simulink library "GFL_Lib"  (R2017a)
settings: Solver=VariableStepAuto  StartTime=0.0  StopTime=10.0  RelTol=1e-3
values from neighbouring files (symbols this model uses):
  Va0 = Vm0*sqrt(2)*Vb1*sin(Theta_Vm0*pi/180)    [Init_LF_L.m]
  Vb0 = Vm0*sqrt(2)*Vb1*sin(Theta_Vm0*pi/180-2*pi/3)    [Init_LF_L.m]
  Vc0 = Vm0*sqrt(2)*Vb1*sin(Theta_Vm0*pi/180+2*pi/3)    [Init_LF_L.m]
  Vm0 = abs(V1)    [Init_LF_L.m]
  Vm0_d = Vvsc0*cos(angle(Vvirt))    [Init_LF_L.m]
  Vm0_q = Vvsc0*sin(angle(Vvirt))    [Init_LF_L.m]
  Vvsc0 = abs(Vvirt)    [Init_LF_L.m]
undefined symbols (not defined in the file or in its folder): Diff_CC_ki, Diff_CC_kp, fb, Ib2, Idcb, Ki_i, Ki_Wdiff_pu, Ki_Wtot_pu, Kp_i, Kp_Rvi_pu, Kp_Wdiff_pu, Kp_Wtot_pu, Lb, Lc_eq, Lc_pu, Lf_pu, Sb, Solver_Time_Step, Vb1, Vb2, Vdcb, VSC01_id0, wb, Zb
undefined symbols (not defined in the file): Carm, Time_Step
libraries: powerlib x90, Control_Lib x57, spsCurrentMeasurementLib x7, simulink x7, spsControlledCurrentSourceLib x6, GFL_Lib x5, Source_Lib x2, eeGeneralControl x2, powerlib_meascontrol x2, GFo_Lib x1
(part 1 of 5)
settings Model: Creator=Frederic_Colas  LastModifiedBy=Frederic_Colas

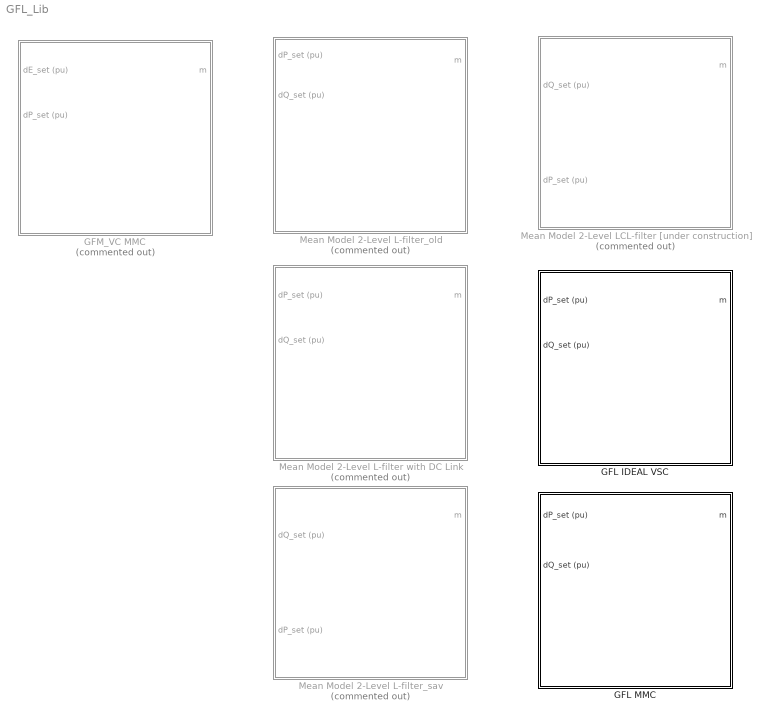
== system GFL_Lib ==
  GFL IDEAL VSC : Subsystem  mask(VSC){fn=50, Sn=1000e6, Pn=1000e6, Udcn=640e3, Output_Delay=100e-6, Un1=320e3, Un2=400e3, m=1, Rt_pu=0.005, Lt_pu=0.15+0.18/2, Lm_pu=500, Rm_pu=500, DC_Link=Perfect DC Source, H_DC=inf, H_DC_sav=inf, wn_PLL=50, zeta_PLL=1, QV=Voltage Control, w_P=5, w_V=10, w_LPF=30, wn_i=4000, zeta_i=1, Kffi=on, Filtre_FF=off, w_ff=4000, Imax=5, Iqmax=5, K_FRT=0, Advanced=on, LFpopup=PQ, P0=0, Q0=0, V0=1, Theta0=0}
      mask prompts: fn "Nominal Frequency (Hz)"; Sn "Nominal Apparent Power (VA)"; Pn "Nominal Power (W)"; Udcn "Nominal DC Voltage (V)"; Output_Delay "Equivalent Ouput Delay (s)"; Un1 "VSC side Nominal Ph-Ph Voltage (V)"; Un2 "Grid side Nominal Ph-Ph Voltage (V)"; m "Transformer's ratio (p.u)"; Rt_pu "R (pu)"; Lt_pu "L (pu)"; Lm_pu "Rm (pu)"; Rm_pu "Lm (pu)"; H_DC "DC Inertia (ms)"; wn_PLL "Bandwidth (rad/s)"; zeta_PLL "Damping Ratio"; QV "Mode"; w_P "Power control bandwidth (rad/s)"; w_V "Voltage control bandwidth (rad/s)"; w_LPF "Low-pass filters bandwidth (rad/s)"; wn_i "Bandwidth (rad/s)"; zeta_i "Damping factor"; Kffi "Feedfoward Enable"; Filtre_FF "Filter of ff enable"; w_ff "Cutoff pulsation (rad/s)"; Imax "Maximum current"; Iqmax "Maximum quadrature current"; K_FRT "LVRT block enabled (1) or disabled (0)"; P0 "Initial Active Power (pu)"; Q0 "Initial Reactive Power (pu)"; V0 "Initial Voltage (pu)"; Theta0 "Initial Angle (°)"
      mask init:
      | Init_Base;
      | dLc_pu = 0;
      | Init_VI;
      | Init_LF_L;
      | Init_GFL;
      settings: OpenFcn=|
      | NameStr = get_param(gcb,'Name');
      | open_system(gcbh, 'Mask');
      | 
      | h2AllOpenDlgs = DAStudio.ToolRoot.getOpenDialogs;
      | 
      | for i=1:length(h2AllOpenDlgs)
      |     try
      |          %disp(h2AllOpenDlgs(i).getSource.getBlock.Name);
      |         Dialog_block_name = h2AllOpenDlgs(i).getSource.getBlock.Name;
      |          %strcmp(Dialog_block_name, NameStr),
      |         if (strcmp(h2AllOpenDlgs(i).getSource.getBlock.Name, NameStr))
      |             iPos = h2AllOpenDlgs(i).position;
      |             h2AllOpenDlgs(i).position = [iPos(1)   iPos(2)   iPos(3)*1.4   iPos(4)];
      |         end
      |     end
      | end
      mask TypeOptions DC_Link: Perfect DC Source | No DC link capacitor | DC link capacitor
      mask Callback DC_Link:
      | % Get the mask parameter values. This is a cell
      | %   array of character vectors.
      | maskStr = get_param(gcb,'DC_Link');
      | p=Simulink.Mask.get(gcb);
      | 
      | % The pop-up menu is the first mask parameter.
      | %   Check the value selected in the pop-up
      | if strcmp(maskStr,'Perfect DC Source'),
      |     % Set the visibility of both parameters on when
      |     %   User-defined is selected in the pop-up.
      |     if strcmp(p.getParameter('H_DC').Visible,'on')
      |         p.getParameter('H_DC_sav').Value=p.getParameter('H_DC').Value;
      |     end
      |     p.getParameter('H_DC').Visible='off';
      |     p.getParameter('H_DC').Value='inf';
      | elseif strcmp(maskStr,'No DC link capacitor'),
      |     if strcmp(p.getParameter('H_DC').Visible,'on')
      |         p.getParameter('H_DC_sav').Value=p.getParameter('H_DC').Value;
      |     end
      |     p.getParameter('H_DC').Visible='off';
      |     p.getParameter('H_DC').Value='0';
      | else
      |     % Set the visibility of both parameters on when
      |     %   User-defined is selected in the pop-up.
      |     p.getParameter('H_DC').Visible='on';
      |     p.getParameter('H_DC').Value=p.getParameter('H_DC_sav').Value;
      | end
      mask TypeOptions QV: Voltage Control | Reactive Power Control
      mask Callback Advanced:
      | % Get the mask parameter values. This is a cell
      | %   array of character vectors.
      | maskStr = get_param(gcb,'Advanced');
      | p=Simulink.Mask.get(gcb);
      | 
      | % The pop-up menu is the first mask parameter.
      | %   Check the value selected in the pop-up
      | if strcmp(maskStr,'on'),
      | 
      |     % Set the visibility of both parameters on when
      |     %   User-defined is selected in the pop-up.
      |     p.getDialogControl('Current_Loop').Visible='on';
      |     %p.getDialogControl('TVI').Visible='on';
      |     %p.getDialogControl('LC_Filter').Visible='on';
      |     p.getDialogControl('Current_Sat').Visible='on';
      |     p.getDialogControl('LVRT').Visible='on';
      | 
      | 
      | else
      | 
      |     % Set the visibility of both parameters on when
      |     %   User-defined is selected in the pop-up.
      |     p.getDialogControl('Current_Loop').Visible='off';
      |     %p.getDialogControl('TVI').Visible='on';
      |     %p.getDialogControl('LC_Filter').Visible='on';
      |     p.getDialogControl('Current_Sat').Visible='off';
      |     p.getDialogControl('LVRT').Visible='off';
      | 
      | end
      mask TypeOptions LFpopup: Swing | PQ | PV
      mask Callback LFpopup:
      | % Get the mask parameter values. This is a cell
      | %   array of character vectors.
      | maskStr = get_param(gcb,'LFpopup');
      | p=Simulink.Mask.get(gcb);
      | 
      | % The pop-up menu is the first mask parameter.
      | %   Check the value selected in the pop-up
      | if strcmp(maskStr,'Swing'),
      | 
      |     % Set the visibility of both parameters on when
      |     %   User-defined is selected in the pop-up.
      |     p.getParameter('P0').Visible='off';
      |     p.getParameter('Q0').Visible='off';
      |     p.getParameter('V0').Visible='on';
      |     p.getParameter('Theta0').Visible='on';
      |     set_param([gcb '/Source_For_LF'],'BusType','swing');
      | 
      | elseif strcmp(maskStr,'PQ'),
      | 
      |     % Set the visibility of both parameters on when
      |     %   User-defined is selected in the pop-up.
      |     p.getParameter('P0').Visible='on';
      |     p.getParameter('Q0').Visible='on';
      |     p.getParameter('V0').Visible='off';
      |     p.getParameter('Theta0').Visible='off';
      |     set_param([gcb '/Source_For_LF'],'BusType','PQ');
      | 
      |     % Turn off the visibility of the Value field
      |     %   when User-defined is not selected.
      | else
      | 
      |     % Set the visibility of both parameters on when
      |     %   User-defined is selected in the pop-up.
      |     p.getParameter('P0').Visible='on';
      |     p.getParameter('Q0').Visible='off';
      |     p.getParameter('V0').Visible='on';
      |     p.getParameter('Theta0').Visible='off';
      |     set_param([gcb '/Source_For_LF'],'BusType','PV');
      | 
      | end
      mask DialogControl Container13 Prompt: PLL
      mask DialogControl Container11 Prompt: Outer loop
      mask DialogControl Current_Loop Prompt: Current Loop
      mask DialogControl Current_Sat Prompt: Current saturations
      mask DialogControl LVRT Prompt: LVRT
      mask DialogControl Control4 Prompt: Initial Operating Point
      mask DialogControl Container24 Prompt: VSC side
      mask DialogControl LF_vsc_str Prompt: V0 = 1.0002 pu, Angle = 0.013461°
      mask DialogControl Container25 Prompt: PCC
      mask DialogControl UpdateLoadflow Prompt: Update Loadflow
      mask DialogControl UpdateLoadflow Callback: LoadFlow_VSC
      mask Display:
      | x1=0.05;
      | y1=0.2;
      | %
      | plot([0.5 0.5]+x1,[0.97,0.8]-y1)
      | plot([0.5 0.32]+x1,[0.80 0.71]-y1)
      | plot([0.32 0.32]+x1,[0.80 0.52]-y1)
      | plot([0.32 0.5]+x1,[0.62 0.52]-y1)
      | plot([0.5 0.5]+x1,[0.52 0.35]-y1)
      | plot([0.45 0.5 0.43]+x1,[0.59 0.52 0.51]-y1)
      | %
      | plot([0.28 0.28]+x1,[0.74 0.58]-y1)
      | plot([0.28 0.20]+x1,[0.66 0.66]-y1)
      | %
      | plot([0.5 0.63]+x1,[0.84 0.84]-y1)
      | plot([0.63 0.63]+x1,[0.84 0.72]-y1)
      | plot([0.63 0.59]+x1,[0.72 0.65]-y1)
      | plot([0.63 0.67]+x1,[0.72 0.65]-y1)
      | plot([0.59 0.67]+x1,[0.65 0.65]-y1)
      | plot([0.63 0.63]+x1,[0.65 0.47]-y1)
      | plot([0.5 0.63]+x1,[0.47 0.47]-y1)
      | plot([0.58 0.67]+x1,[0.72 0.72]-y1)
      | %
      | color('blue')
      | text(0.3,0.10,'L-Filter GFL')
      | 
      | port_label('input',1,'\DeltaP (pu)','texmode','on');
      | port_label('input',2,'\DeltaQ (pu)','texmode','on');
      | port_label('output',1,'m');
      | port_label('rconn',1,'A');
      | port_label('rconn',2,'B');
      | port_label('rconn',3,'C');
      | port_label('lconn',1,'+');
      | port_label('lconn',2,'-');
  GFL MMC : Subsystem  mask(VSC){fn=50, Sn=1e9, Pn=1e9, Udcn=640e3, Output_Delay=100e-6, Un1=320e3, Un2=400e3, m=1, Rt_pu=0.005, Lt_pu=0.15, Lm_pu=500, Rm_pu=500, Larm_pu=0.18, Rarm_pu=0.005, nSM=0, Hc=40, wn_PLL=50, zeta_PLL=1, QV=Voltage Control, w_P=5, w_V=50, w_LPF=1000, wn_i=300, zeta_i=1, Kffi=on, Filtre_FF=on, w_ff=4000, Imax=5, Iqmax=5, K_FRT=0, MMC_Control_Type=CCSC, Diff_CC_fn=0, Diff_CC_zeta=0, fn_Wtot=0, zeta_Wtot=0, fn_Wdiff=0, zeta_Wdiff=0, Advanced=off, LFpopup=PQ, P0=0, Q0=0, V0=1, Theta0=0}
      mask prompts: fn "Nominal Frequency (Hz)"; Sn "Nominal Apparent Power (VA)"; Pn "Nominal Power (W)"; Udcn "Nominal DC Voltage (V)"; Output_Delay "Equivalent Ouput Delay (s)"; Un1 "VSC side Nominal Ph-Ph Voltage (V)"; Un2 "Grid side Nominal Ph-Ph Voltage (V)"; m "Transformer's ratio (p.u)"; Rt_pu "R (pu)"; Lt_pu "L (pu)"; Lm_pu "Rm (pu)"; Rm_pu "Lm (pu)"; Larm_pu "Arm Inductance (pu)"; Rarm_pu "Arm Resistance (pu)"; nSM "Sub-Modules number"; Hc "Hc (ms)"; wn_PLL "Bandwidth (rad/s)"; zeta_PLL "Damping Ratio"; QV "Mode"; w_P "Power control bandwidth (rad/s)"; w_V "Voltage control bandwidth (rad/s)"; w_LPF "Low-pass filters bandwidth (rad/s)"; wn_i "Bandwidth (rad/s)"; zeta_i "Damping factor"; Kffi "Feedfoward Enable"; Filtre_FF "Filter of ff enable"; w_ff "Cutoff frequency (rad/s)"; Imax "Maximum current"; Iqmax "Maximum quadrature current"; K_FRT "LVRT block enabled (1) or disabled (0)"; MMC_Control_Type "Controller Type"; Diff_CC_fn "Bandwidth (Hz)"; Diff_CC_zeta "Damping"; fn_Wtot "Bandwidth (Hz)"; zeta_Wtot "Damping"; fn_Wdiff "Bandwidth (Hz)"; zeta_Wdiff "Damping"; P0 "Initial Active Power (pu)"; Q0 "Initial Reactive Power (pu)"; V0 "Initial Voltage (pu)"; Theta0 "Initial Angle (°)"
      mask init:
      | Init_Base;
      | dLc_pu = 0;
      | Init_VI_mmc;
      | Init_MMC;
      | Init_LF_MMC;
      | Init_GFL;
      settings: OpenFcn=|
      | NameStr = get_param(gcb,'Name');
      | open_system(gcbh, 'Mask');
      | 
      | h2AllOpenDlgs = DAStudio.ToolRoot.getOpenDialogs;
      | 
      | for i=1:length(h2AllOpenDlgs)
      |     try
      |          %disp(h2AllOpenDlgs(i).getSource.getBlock.Name);
      |         Dialog_block_name = h2AllOpenDlgs(i).getSource.getBlock.Name;
      |          %strcmp(Dialog_block_name, NameStr),
      |         if (strcmp(h2AllOpenDlgs(i).getSource.getBlock.Name, NameStr))
      |             iPos = h2AllOpenDlgs(i).position;
      |             h2AllOpenDlgs(i).position = [iPos(1)   iPos(2)   iPos(3)*1.4   iPos(4)];
      |         end
      |     end
      | end
      mask TypeOptions QV: Voltage Control | Reactive Power Control
      mask TypeOptions MMC_Control_Type: CCSC | Energy Based
      mask Callback MMC_Control_Type:
      | % Get the mask parameter values. This is a cell
      | %   array of character vectors.
      | maskStr = get_param(gcb,'MMC_Control_Type');
      | p=Simulink.Mask.get(gcb);
      | 
      | % The pop-up menu is the first mask parameter.
      | %   Check the value selected in the pop-up
      | if strcmp(maskStr,'CCSC'),
      | 
      |     % Set the visibility of both parameters on when
      |     %   User-defined is selected in the pop-up.
      |     p.getDialogControl('Diff_CC').Visible='on';
      |     %p.getDialogControl('TVI').Visible='on';
      |     %p.getDialogControl('LC_Filter').Visible='on';
      |     p.getDialogControl('Wtot_C').Visible='off';
      |     p.getDialogControl('Wdiff_C').Visible='off';
      |     %p.getDialogControl('Param_Strat_3').Visible='off';
      | 
      | 
      | else
      | 
      |     % Set the visibility of both parameters on when
      |     %   User-defined is selected in the pop-up.
      |     p.getDialogControl('Diff_CC').Visible='on';
      |     %p.getDialogControl('TVI').Visible='on';
      |     %p.getDialogControl('LC_Filter').Visible='on';
      |     p.getDialogControl('Wtot_C').Visible='on';
      |     p.getDialogControl('Wdiff_C').Visible='on';
      |     %p.getDialogControl('Param_Strat_3').Visible='off';
      | 
      | end
      mask Callback Advanced:
      | % Get the mask parameter values. This is a cell
      | %   array of character vectors.
      | maskStr = get_param(gcb,'Advanced');
      | p=Simulink.Mask.get(gcb);
      | 
      | % The pop-up menu is the first mask parameter.
      | %   Check the value selected in the pop-up
      | if strcmp(maskStr,'on'),
      | 
      |     % Set the visibility of both parameters on when
      |     %   User-defined is selected in the pop-up.
      |     p.getDialogControl('Current_Loop').Visible='on';
      |     %p.getDialogControl('TVI').Visible='on';
      |     %p.getDialogControl('LC_Filter').Visible='on';
      |     p.getDialogControl('Current_Sat').Visible='on';
      |     p.getDialogControl('LVRT').Visible='on';
      |     p.getDialogControl('MMC_Control').Visible='on';
      | 
      | 
      | else
      | 
      |     % Set the visibility of both parameters on when
      |     %   User-defined is selected in the pop-up.
      |     p.getDialogControl('Current_Loop').Visible='off';
      |     %p.getDialogControl('TVI').Visible='on';
      |     %p.getDialogControl('LC_Filter').Visible='on';
      |     p.getDialogControl('Current_Sat').Visible='off';
      |     p.getDialogControl('LVRT').Visible='off';
      |     p.getDialogControl('MMC_Control').Visible='off';
      | 
      | end
      mask TypeOptions LFpopup: Swing | PQ | PV
      mask Callback LFpopup:
      | % Get the mask parameter values. This is a cell
      | %   array of character vectors.
      | maskStr = get_param(gcb,'LFpopup');
      | p=Simulink.Mask.get(gcb);
      | 
      | % The pop-up menu is the first mask parameter.
      | %   Check the value selected in the pop-up
      | if strcmp(maskStr,'Swing'),
      | 
      |     % Set the visibility of both parameters on when
      |     %   User-defined is selected in the pop-up.
      |     p.getParameter('P0').Visible='off';
      |     p.getParameter('Q0').Visible='off';
      |     p.getParameter('V0').Visible='on';
      |     p.getParameter('Theta0').Visible='on';
      |     set_param([gcb '/Source_For_LF'],'BusType','swing');
      | 
      | elseif strcmp(maskStr,'PQ'),
      | 
      |     % Set the visibility of both parameters on when
      |     %   User-defined is selected in the pop-up.
      |     p.getParameter('P0').Visible='on';
      |     p.getParameter('Q0').Visible='on';
      |     p.getParameter('V0').Visible='off';
      |     p.getParameter('Theta0').Visible='off';
      |     set_param([gcb '/Source_For_LF'],'BusType','PQ');
      | 
      |     % Turn off the visibility of the Value field
      |     %   when User-defined is not selected.
      | else
      | 
      |     % Set the visibility of both parameters on when
      |     %   User-defined is selected in the pop-up.
      |     p.getParameter('P0').Visible='on';
      |     p.getParameter('Q0').Visible='off';
      |     p.getParameter('V0').Visible='on';
      |     p.getParameter('Theta0').Visible='off';
      |     set_param([gcb '/Source_For_LF'],'BusType','PV');
      | 
      | end
      mask DialogControl Container13 Prompt: PLL
      mask DialogControl Container11 Prompt: Outer loop
      mask DialogControl Current_Loop Prompt: Current Loop
      mask DialogControl Current_Sat Prompt: Current saturations
      mask DialogControl LVRT Prompt: LVRT
      mask DialogControl MMC_Control Prompt: MMC Controller
      mask DialogControl Diff_CC Prompt: Differential Current Controller
      mask DialogControl Wtot_C Prompt: Wtot Controller
      mask DialogControl Wdiff_C Prompt: Wdiff Controller
      mask DialogControl Control4 Prompt: Initial Operating Point
      mask DialogControl Container24 Prompt: VSC side
      mask DialogControl LF_vsc_str Prompt: V0 = 1.0003 pu, Angle = 0.018328°
      mask DialogControl Container25 Prompt: PCC
      mask DialogControl UpdateLoadflow Prompt: Update Loadflow
      mask DialogControl UpdateLoadflow Callback: LoadFlow_VSC
      mask Display:
      | % Q1
      | x1=-0.07;
      | y1=+0.03;
      | plot([0.4 0.4]+x1,[0.90,0.80]+y1)
      | plot([0.4 0.33]+x1,[0.80 0.74]+y1)
      | plot([0.33 0.33]+x1,[0.78 0.66]+y1)
      | plot([0.33 0.4]+x1,[0.70 0.64]+y1)
      | plot([0.4 0.4]+x1,[0.64 0.55]+y1)
      | plot([0.38 0.40 0.35]+x1,[0.68 0.64 0.64]+y1)
      | plot([0.30 0.30]+x1,[0.74 0.7]+y1)
      | plot([0.29 0.27]+x1,[0.72 0.72]+y1)
      | % Q2
      | y1=y1-0.51;
      | plot([0.4 0.4]+x1,[0.90,0.80]+y1)
      | plot([0.4 0.33]+x1,[0.80 0.74]+y1)
      | plot([0.33 0.33]+x1,[0.78 0.66]+y1)
      | plot([0.33 0.4]+x1,[0.70 0.64]+y1)
      | plot([0.4 0.4]+x1,[0.64 0.55]+y1)
      | plot([0.39 0.40 0.35]+x1,[0.68 0.64 0.64]+y1)
      | plot([0.30 0.30]+x1,[0.75 0.7]+y1)
      | plot([0.29 0.27]+x1,[0.72 0.72]+y1)
      | % Q3
      | y1=y1+0.51;
      | x1=x1+0.22+0.1;
      | plot([0.4 0.4]+x1,[0.90,0.80]+y1)
      | plot([0.4 0.33]+x1,[0.80 0.74]+y1)
      | plot([0.33 0.33]+x1,[0.78 0.66]+y1)
      | plot([0.33 0.4]+x1,[0.70 0.64]+y1)
      | plot([0.4 0.4]+x1,[0.64 0.55]+y1)
      | plot([0.39 0.41 0.34]+x1,[0.68 0.64 0.64]+y1)
      | plot([0.30 0.30]+x1,[0.75 0.7]+y1)
      | plot([0.29 0.27]+x1,[0.72 0.72]+y1)
      | % Q4
      | y1=y1-0.51;
      | x1=x1;
      | plot([0.4 0.4]+x1,[0.90,0.80]+y1)
      | plot([0.4 0.33]+x1,[0.80 0.74]+y1)
      | plot([0.33 0.33]+x1,[0.78 0.66]+y1)
      | plot([0.33 0.4]+x1,[0.70 0.64]+y1)
      | plot([0.4 0.4]+x1,[0.64 0.55]+y1)
      | plot([0.39 0.41 0.34]+x1,[0.68 0.64 0.64]+y1)
      | plot([0.30 0.30]+x1,[0.75 0.7]+y1)
      | plot([0.29 0.26]+x1,[0.72 0.72]+y1)
      | %
      | x1=-0.05;
      | y1=+0.03;
      | plot([0.90 0.40]+x1,[0.9 0.9]+y1)
      | plot([0.90 0.40]+x1,[0.04 0.04]+y1)
      | %
      | 
      | plot([0.69 0.42]+x1,[0.4 0.4]+y1)
      | plot([0.38 0.22]+x1,[0.52 0.52]+y1)
      | plot([0.22 0.22]+x1,[0.52 0.54]+y1)
      | plot([0.22 0.22]+x1,[0.56 0.58]+y1)
      | plot([0.22 0.22]+x1,[0.60 0.63]+y1)
      | %
      | plot([0.35 0.22]+x1,[0.4 0.4]+y1)
      | plot([0.22 0.22]+x1,[0.4 0.37]+y1)
      | plot([0.22 0.22]+x1,[0.4 0.37]+y1)
      | plot([0.22 0.22]+x1,[0.35 0.32]+y1)
      | plot([0.22 0.22]+x1,[0.30 0.27]+y1)
      | %
      | plot([0.38 0.38]+x1,[ 0.55 0.38]+y1)
      | plot([0.7 0.7]+x1,[0.55 0.3]+y1)
      | %
      | % D1
      | x1=-0.07;
      | y1=+0.03;
      | plot([0.4 0.45]+x1,[0.84,0.84]+y1)
      | plot([0.45 0.45]+x1,[0.84,0.75]+y1)
      | plot([0.45 0.41]+x1,[0.75,0.72]+y1)
      | plot([0.45 0.48]+x1,[0.75,0.72]+y1)
      | plot([0.41 0.48]+x1,[0.72,0.72]+y1)
      | plot([0.45 0.45]+x1,[0.72,0.6]+y1)
      | plot([0.4 0.45]+x1,[0.6,0.6]+y1)
      | % D2
      | x1=x1+0.22+0.1;
      | plot([0.4 0.45]+x1,[0.84,0.84]+y1)
      | plot([0.45 0.45]+x1,[0.84,0.75]+y1)
      | plot([0.45 0.43]+x1,[0.75,0.72]+y1)
      | plot([0.45 0.48]+x1,[0.75,0.72]+y1)
      | %
      | plot([0.43 0.48]+x1,[0.72,0.72]+y1)
      | plot([0.45 0.45]+x1,[0.72,0.6]+y1)
      | plot([0.4 0.45]+x1,[0.6,0.6]+y1)
      | % D3
      | x1=x1-0.22-0.1;
      | y1=y1-0.5;
      | plot([0.4 0.45]+x1,[0.84,0.84]+y1)
      | plot([0.45 0.45]+x1,[0.84,0.75]+y1)
      | plot([0.45 0.41]+x1,[0.75,0.72]+y1)
      | plot([0.45 0.48]+x1,[0.75,0.72]+y1)
      | plot([0.41 0.48]+x1,[0.72,0.72]+y1)
      | plot([0.45 0.45]+x1,[0.72,0.6]+y1)
      | plot([0.4 0.45]+x1,[0.6,0.6]+y1)
      | % D4
      | x1=x1+0.22+0.1;
      | plot([0.4 0.45]+x1,[0.84,0.84]+y1)
      | plot([0.45 0.45]+x1,[0.84,0.75]+y1)
      | plot([0.45 0.43]+x1,[0.75,0.72]+y1)
      | plot([0.45 0.48]+x1,[0.75,0.72]+y1)
      | plot([0.43 0.48]+x1,[0.72,0.72]+y1)
      | plot([0.45 0.45]+x1,[0.72,0.6]+y1)
      | plot([0.40 0.45]+x1,[0.6,0.6]+y1)
      | color('blue');
      | disp('MMC GFL');
      | port_label('input',1,'\DeltaE (pu)','texmode','on');
      | port_label('input',2,'\DeltaP (pu)','texmode','on');
      | port_label('output',1,'m');
      | port_label('rconn',1,'A');
      | port_label('rconn',2,'B');
      | port_label('rconn',3,'C');
      | port_label('lconn',1,'+');
      | port_label('lconn',2,'-');
  GFM_VC MMC : Subsystem  Commented=on  mask(VSC){fn=50, Sn=1000e6, Pn=1000e6, Udcn=640e3, Output_Delay=100e-6, Un1=320e3, Un2=400e3, Rt_pu=0.005, Lt_pu=0.15, Lm_pu=500, Rm_pu=500, Larm_pu=0.18, Rarm_pu=0.005, nSM=0, Hc=40, DC_source=on, wn_PLL=50, zeta_PLL=1, Val_Freq_Support=off, R_percent=4, dLc_pu=0, Rv=0.009, W_TVR=60, I_max_pu=2, Tr_I_max=10, I_Max_TVI_pu=2, DX_DR=5, MMC_Control_Type=CCSC, Diff_CC_fn=200, Diff_CC_zeta=1, fn_Wtot=3, zeta_Wtot=1, fn_Wdiff=3, zeta_Wdiff=1, Advanced=on, gainpopup=With Inertia, wn_Inertia_Less=5, Param_Inertia=PI, H_GFo=5, zeta_GFo=1, LFpopup=PQ, P0=0, Q0=0, V0=1, Theta0=9.4519e-16}
      mask prompts: fn "Nominal Frequency (Hz)"; Sn "Nominal Apparent Power (VA)"; Pn "Nominal Power (W)"; Udcn "Nominal DC Voltage (V)"; Output_Delay "Equivalent Output Delay (s)"; Un1 "VSC side Nominal Ph-Ph Voltage (V)"; Un2 "Grid side Nominal Ph-Ph Voltage (V)"; Rt_pu "R (pu)"; Lt_pu "L (pu)"; Lm_pu "Rm (pu)"; Rm_pu "Lm (pu)"; Larm_pu "Arm Inductance (pu)"; Rarm_pu "Arm Resistance (pu)"; nSM "Sub-Modules number"; Hc "Hc (ms)"; DC_source "Perfect DC source"; wn_PLL "Bandwidth (rad/s)"; zeta_PLL "Damping Ratio"; Val_Freq_Support "Frequency Support"; R_percent "Droop Gain (%)"; dLc_pu "Additional Virtual Impedance (pu)"; Rv "Damping Resistance (Rv)"; W_TVR "Dr filter"; I_max_pu "I max (pu)"; Tr_I_max "Current Loop time response (ms)"; I_Max_TVI_pu "Current Threshold (pu)"; MMC_Control_Type "Controller Type"; Diff_CC_fn "Bandwidth (Hz)"; Diff_CC_zeta "Damping"; fn_Wtot "Bandwidth (Hz)"; zeta_Wtot "Damping"; fn_Wdiff "Bandwidth (Hz)"; zeta_Wdiff "Damping"; gainpopup "Strategy"; wn_Inertia_Less "Bandwidth (rad/s)"; H_GFo "Inertia H (s)"; zeta_GFo "Damping Ratio"; P0 "Initial Active Power (pu)"; Q0 "Initial Reactive Power (pu)"; V0 "Initial Voltage (pu)"; Theta0 "Initial Angle (°)"
      mask init:
      | Init_Base;
      | Init_VI;
      | Init_MMC;
      | Init_LF_MMC;
      | Init_GFM;
      settings: OpenFcn=|
      | NameStr = get_param(gcb,'Name');
      | open_system(gcbh, 'Mask');
      | 
      | h2AllOpenDlgs = DAStudio.ToolRoot.getOpenDialogs;
      | 
      | for i=1:length(h2AllOpenDlgs)
      |     try
      |          %disp(h2AllOpenDlgs(i).getSource.getBlock.Name);
      |         Dialog_block_name = h2AllOpenDlgs(i).getSource.getBlock.Name;
      |          %strcmp(Dialog_block_name, NameStr),
      |         if (strcmp(h2AllOpenDlgs(i).getSource.getBlock.Name, NameStr))
      |             iPos = h2AllOpenDlgs(i).position;
      |             h2AllOpenDlgs(i).position = [iPos(1)   iPos(2)   iPos(3)*1.4   iPos(4)];
      |         end
      |     end
      | end
      mask TypeOptions MMC_Control_Type: CCSC | Energy Based
      mask Callback MMC_Control_Type:
      | % Get the mask parameter values. This is a cell
      | %   array of character vectors.
      | maskStr = get_param(gcb,'MMC_Control_Type');
      | p=Simulink.Mask.get(gcb);
      | 
      | % The pop-up menu is the first mask parameter.
      | %   Check the value selected in the pop-up
      | if strcmp(maskStr,'CCSC'),
      | 
      |     % Set the visibility of both parameters on when
      |     %   User-defined is selected in the pop-up.
      |     p.getDialogControl('Diff_CC').Visible='on';
      |     %p.getDialogControl('TVI').Visible='on';
      |     %p.getDialogControl('LC_Filter').Visible='on';
      |     p.getDialogControl('Wtot_C').Visible='off';
      |     p.getDialogControl('Wdiff_C').Visible='off';
      |     %p.getDialogControl('Param_Strat_3').Visible='off';
      | 
      | 
      | else
      | 
      |     % Set the visibility of both parameters on when
      |     %   User-defined is selected in the pop-up.
      |     p.getDialogControl('Diff_CC').Visible='on';
      |     %p.getDialogControl('TVI').Visible='on';
      |     %p.getDialogControl('LC_Filter').Visible='on';
      |     p.getDialogControl('Wtot_C').Visible='on';
      |     p.getDialogControl('Wdiff_C').Visible='on';
      |     %p.getDialogControl('Param_Strat_3').Visible='off';
      | 
      | end
      mask Callback Advanced:
      | % Get the mask parameter values. This is a cell
      | %   array of character vectors.
      | maskStr = get_param(gcb,'Advanced');
      | p=Simulink.Mask.get(gcb);
      | 
      | % The pop-up menu is the first mask parameter.
      | %   Check the value selected in the pop-up
      | if strcmp(maskStr,'on'),
      | 
      |     % Set the visibility of both parameters on when
      |     %   User-defined is selected in the pop-up.
      |     p.getDialogControl('TVR').Visible='on';
      |     %p.getDialogControl('TVI').Visible='on';
      |     %p.getDialogControl('LC_Filter').Visible='on';
      |     p.getDialogControl('Current_Sat').Visible='on';
      |     p.getDialogControl('MMC_Control').Visible='on';
      |     %p.getDialogControl('Param_Strat_3').Visible='off';
      | 
      | 
      | else
      | 
      |     % Set the visibility of both parameters on when
      |     %   User-defined is selected in the pop-up.
      |     p.getDialogControl('TVR').Visible='off';
      |     %p.getDialogControl('TVI').Visible='off';
      |     %p.getDialogControl('LC_Filter').Visible='off';
      |     p.getDialogControl('Current_Sat').Visible='off';
      |     p.getDialogControl('MMC_Control').Visible='off';
      |     %p.getDialogControl('Param_Strat_3').Visible='off';
      | 
      | end
      mask TypeOptions gainpopup: Inertia Less | With Inertia
      mask Callback gainpopup:
      | % Get the mask parameter values. This is a cell
      | %   array of character vectors.
      | maskStr = get_param(gcb,'gainpopup');
      | p=Simulink.Mask.get(gcb);
      | 
      | % The pop-up menu is the first mask parameter.
      | %   Check the value selected in the pop-up
      | if strcmp(maskStr,'Inertia Less'),
      | 
      |     % Set the visibility of both parameters on when
      |     %   User-defined is selected in the pop-up.
      |     p.getDialogControl('No_Inertia').Visible='on';
      |     p.getDialogControl('Inertia').Visible='off';
      |     %p.getDialogControl('Param_Strat_3').Visible='off';
      | 
      | 
      | elseif strcmp(maskStr,'With Inertia'),
      | 
      |     % Set the visibility of both parameters on when
      |     %   User-defined is selected in the pop-up.
      |     p.getDialogControl('No_Inertia').Visible='off';
      |     p.getDialogControl('Inertia').Visible='on';
      |     %p.getDialogControl('Param_Strat_3').Visible='off';
      | 
      | 
      |     % Turn off the visibility of the Value field
      |     %   when User-defined is not selected.
      | 
      | else
      | 
      |     % Set the visibility of both parameters on when
      |     %   User-defined is selected in the pop-up.
      |     p.getDialogControl('No_Inertia').Visible='off';
      |     p.getDialogControl('Inertia').Visible='off';
      |     %p.getDialogControl('Param_Strat_3').Visible='off';
      | 
      | end
      mask TypeOptions Param_Inertia: VSM | PI
      mask TypeOptions LFpopup: Swing | PQ | PV
      mask Callback LFpopup:
      | % Get the mask parameter values. This is a cell
      | %   array of character vectors.
      | maskStr = get_param(gcb,'LFpopup');
      | p=Simulink.Mask.get(gcb);
      | 
      | % The pop-up menu is the first mask parameter.
      | %   Check the value selected in the pop-up
      | if strcmp(maskStr,'Swing'),
      | 
      |     % Set the visibility of both parameters on when
      |     %   User-defined is selected in the pop-up.
      |     p.getParameter('P0').Visible='off';
      |     p.getParameter('Q0').Visible='off';
      |     p.getParameter('V0').Visible='on';
      |     p.getParameter('Theta0').Visible='on';
      |     set_param([gcb '/Source_For_LF'],'BusType','swing');
      | 
      | elseif strcmp(maskStr,'PQ'),
      | 
      |     % Set the visibility of both parameters on when
      |     %   User-defined is selected in the pop-up.
      |     p.getParameter('P0').Visible='on';
      |     p.getParameter('Q0').Visible='on';
      |     p.getParameter('V0').Visible='off';
      |     p.getParameter('Theta0').Visible='off';
      |     set_param([gcb '/Source_For_LF'],'BusType','PQ');
      | 
      |     % Turn off the visibility of the Value field
      |     %   when User-defined is not selected.
      | else
      | 
      |     % Set the visibility of both parameters on when
      |     %   User-defined is selected in the pop-up.
      |     p.getParameter('P0').Visible='on';
      |     p.getParameter('Q0').Visible='off';
      |     p.getParameter('V0').Visible='on';
      |     p.getParameter('Theta0').Visible='off';
      |     set_param([gcb '/Source_For_LF'],'BusType','PV');
      | 
      | end
      mask DialogControl Container21 Prompt: Output Transformer
      mask DialogControl Container22 Prompt: Sub-Modules & Arm
      mask DialogControl Container13 Prompt: PLL
      mask DialogControl Container14 Prompt: Frequency Support
      mask DialogControl VI Prompt: Virtual Impedance
      mask DialogControl TVR Prompt: Transient Virtual Resistor
      mask DialogControl Current_Sat Prompt: Current Limitation
      mask DialogControl MMC_Control Prompt: MMC Controller
      mask DialogControl Diff_CC Prompt: Differential Current Controller
      mask DialogControl Wtot_C Prompt: Wtot Controller
      mask DialogControl Wdiff_C Prompt: Wdiff Controller
      mask DialogControl Control4 Prompt: Initial Operating Point
      mask DialogControl Container24 Prompt: VSC side
      mask DialogControl LF_vsc_str Prompt: V0 = 1.0003 pu, Angle = 0.018328°
      mask DialogControl Container25 Prompt: PCC
      mask DialogControl UpdateLoadflow Prompt: Update Loadflow
      mask DialogControl UpdateLoadflow Callback: LoadFlow_VSC
      mask Display:
      | % Q1
      | x1=-0.07;
      | y1=+0.03;
      | plot([0.4 0.4]+x1,[0.90,0.80]+y1)
      | plot([0.4 0.33]+x1,[0.80 0.74]+y1)
      | plot([0.33 0.33]+x1,[0.78 0.66]+y1)
      | plot([0.33 0.4]+x1,[0.70 0.64]+y1)
      | plot([0.4 0.4]+x1,[0.64 0.55]+y1)
      | plot([0.38 0.40 0.35]+x1,[0.68 0.64 0.64]+y1)
      | plot([0.30 0.30]+x1,[0.74 0.7]+y1)
      | plot([0.29 0.27]+x1,[0.72 0.72]+y1)
      | % Q2
      | y1=y1-0.51;
      | plot([0.4 0.4]+x1,[0.90,0.80]+y1)
      | plot([0.4 0.33]+x1,[0.80 0.74]+y1)
      | plot([0.33 0.33]+x1,[0.78 0.66]+y1)
      | plot([0.33 0.4]+x1,[0.70 0.64]+y1)
      | plot([0.4 0.4]+x1,[0.64 0.55]+y1)
      | plot([0.39 0.40 0.35]+x1,[0.68 0.64 0.64]+y1)
      | plot([0.30 0.30]+x1,[0.75 0.7]+y1)
      | plot([0.29 0.27]+x1,[0.72 0.72]+y1)
      | % Q3
      | y1=y1+0.51;
      | x1=x1+0.22+0.1;
      | plot([0.4 0.4]+x1,[0.90,0.80]+y1)
      | plot([0.4 0.33]+x1,[0.80 0.74]+y1)
      | plot([0.33 0.33]+x1,[0.78 0.66]+y1)
      | plot([0.33 0.4]+x1,[0.70 0.64]+y1)
      | plot([0.4 0.4]+x1,[0.64 0.55]+y1)
      | plot([0.39 0.41 0.34]+x1,[0.68 0.64 0.64]+y1)
      | plot([0.30 0.30]+x1,[0.75 0.7]+y1)
      | plot([0.29 0.27]+x1,[0.72 0.72]+y1)
      | % Q4
      | y1=y1-0.51;
      | x1=x1;
      | plot([0.4 0.4]+x1,[0.90,0.80]+y1)
      | plot([0.4 0.33]+x1,[0.80 0.74]+y1)
      | plot([0.33 0.33]+x1,[0.78 0.66]+y1)
      | plot([0.33 0.4]+x1,[0.70 0.64]+y1)
      | plot([0.4 0.4]+x1,[0.64 0.55]+y1)
      | plot([0.39 0.41 0.34]+x1,[0.68 0.64 0.64]+y1)
      | plot([0.30 0.30]+x1,[0.75 0.7]+y1)
      | plot([0.29 0.26]+x1,[0.72 0.72]+y1)
      | %
      | x1=-0.05;
      | y1=+0.03;
      | plot([0.90 0.40]+x1,[0.9 0.9]+y1)
      | plot([0.90 0.40]+x1,[0.04 0.04]+y1)
      | %
      | 
      | plot([0.69 0.42]+x1,[0.4 0.4]+y1)
      | plot([0.38 0.22]+x1,[0.52 0.52]+y1)
      | plot([0.22 0.22]+x1,[0.52 0.54]+y1)
      | plot([0.22 0.22]+x1,[0.56 0.58]+y1)
      | plot([0.22 0.22]+x1,[0.60 0.63]+y1)
      | %
      | plot([0.35 0.22]+x1,[0.4 0.4]+y1)
      | plot([0.22 0.22]+x1,[0.4 0.37]+y1)
      | plot([0.22 0.22]+x1,[0.4 0.37]+y1)
      | plot([0.22 0.22]+x1,[0.35 0.32]+y1)
      | plot([0.22 0.22]+x1,[0.30 0.27]+y1)
      | %
      | plot([0.38 0.38]+x1,[ 0.55 0.38]+y1)
      | plot([0.7 0.7]+x1,[0.55 0.3]+y1)
      | %
      | % D1
      | x1=-0.07;
      | y1=+0.03;
      | plot([0.4 0.45]+x1,[0.84,0.84]+y1)
      | plot([0.45 0.45]+x1,[0.84,0.75]+y1)
      | plot([0.45 0.41]+x1,[0.75,0.72]+y1)
      | plot([0.45 0.48]+x1,[0.75,0.72]+y1)
      | plot([0.41 0.48]+x1,[0.72,0.72]+y1)
      | plot([0.45 0.45]+x1,[0.72,0.6]+y1)
      | plot([0.4 0.45]+x1,[0.6,0.6]+y1)
      | % D2
      | x1=x1+0.22+0.1;
      | plot([0.4 0.45]+x1,[0.84,0.84]+y1)
      | plot([0.45 0.45]+x1,[0.84,0.75]+y1)
      | plot([0.45 0.43]+x1,[0.75,0.72]+y1)
      | plot([0.45 0.48]+x1,[0.75,0.72]+y1)
      | %
      | plot([0.43 0.48]+x1,[0.72,0.72]+y1)
      | plot([0.45 0.45]+x1,[0.72,0.6]+y1)
      | plot([0.4 0.45]+x1,[0.6,0.6]+y1)
      | % D3
      | x1=x1-0.22-0.1;
      | y1=y1-0.5;
      | plot([0.4 0.45]+x1,[0.84,0.84]+y1)
      | plot([0.45 0.45]+x1,[0.84,0.75]+y1)
      | plot([0.45 0.41]+x1,[0.75,0.72]+y1)
      | plot([0.45 0.48]+x1,[0.75,0.72]+y1)
      | plot([0.41 0.48]+x1,[0.72,0.72]+y1)
      | plot([0.45 0.45]+x1,[0.72,0.6]+y1)
      | plot([0.4 0.45]+x1,[0.6,0.6]+y1)
      | % D4
      | x1=x1+0.22+0.1;
      | plot([0.4 0.45]+x1,[0.84,0.84]+y1)
      | plot([0.45 0.45]+x1,[0.84,0.75]+y1)
      | plot([0.45 0.43]+x1,[0.75,0.72]+y1)
      | plot([0.45 0.48]+x1,[0.75,0.72]+y1)
      | plot([0.43 0.48]+x1,[0.72,0.72]+y1)
      | plot([0.45 0.45]+x1,[0.72,0.6]+y1)
      | plot([0.40 0.45]+x1,[0.6,0.6]+y1)
      | color('blue');
      | disp('MMC GFL');
      | port_label('input',1,'\DeltaE (pu)','texmode','on');
      | port_label('input',2,'\DeltaP (pu)','texmode','on');
      | port_label('output',1,'m');
      | port_label('rconn',1,'A');
      | port_label('rconn',2,'B');
      | port_label('rconn',3,'C');
      | port_label('lconn',1,'+');
      | port_label('lconn',2,'-');
  Mean Model 2-Level L-filter with DC Link : Subsystem  Commented=on  mask(VSC){fn=50.0, Sn=1e9, Pn=1e9, Udcn=640e3, Time_Step=Time_Step, Un1=320e3, Un2=400e3, m=1, Rt_pu=0.005, Lt_pu=0.15, Lm_pu=inf, Rm_pu=inf, H_DC=40, Tr_PLL=100, wn_i=1500, zeta_i=0.7, Kffi=on, Filtre_FF=off, w_ff=1000, QV=Reactive Power Control, w_P=10, w_V=50, w_LPF=4000, Imax=5, Iqmax=5, K_FRT=0, LFpopup=PQ, P0=0, Q0=0, V0=1.0108, Theta0=0.4912}
      mask prompts: fn "Nominal Frequency (Hz)"; Sn "Nominal Apparent Power (VA)"; Pn "Nominal Power (W)"; Udcn "Nominal DC Voltage (V)"; Time_Step "Sample Time (s)"; Un1 "VSC side Nominal Ph-Ph Voltage (V)"; Un2 "Grid side Nominal Ph-Ph Voltage (V)"; m "Transformer's ratio (p.u)"; Rt_pu "R (pu)"; Lt_pu "L (pu)"; Lm_pu "Rm (pu)"; Rm_pu "Lm (pu)"; H_DC "DC inertias (ms)"; Tr_PLL "Time response (ms)"; wn_i "Bandwidth (rad/s)"; zeta_i "Damping factor"; Kffi "Feedfoward Enable"; Filtre_FF "Filter of ff enable"; w_ff "Cutoff frequency (rad/s)"; QV "Mode"; w_P "Power control bandwidth"; w_V "Voltage control bandwidth"; w_LPF "Low-pass filters bandwidth"; Imax "Maximum current"; Iqmax "Maximum quadrature current"; K_FRT "LVRT block enabled (1) or disabled (0)"; P0 "Initial Active Power (pu)"; Q0 "Initial Reactive Power (pu)"; V0 "Initial Voltage (pu)"; Theta0 "Initial Angle (°)"
      mask init:
      | Init_Base;
      | Init_LF_L;
      | Init_GFL;
      | Init_Cdc;
      settings: OpenFcn=|
      | NameStr = get_param(gcb,'Name');
      | open_system(gcbh, 'Mask');
      | 
      | h2AllOpenDlgs = DAStudio.ToolRoot.getOpenDialogs;
      | 
      | for i=1:length(h2AllOpenDlgs)
      |     try
      |          %disp(h2AllOpenDlgs(i).getSource.getBlock.Name);
      |         Dialog_block_name = h2AllOpenDlgs(i).getSource.getBlock.Name;
      |          %strcmp(Dialog_block_name, NameStr),
      |         if (strcmp(h2AllOpenDlgs(i).getSource.getBlock.Name, NameStr))
      |             iPos = h2AllOpenDlgs(i).position;
      |             h2AllOpenDlgs(i).position = [iPos(1)   iPos(2)   iPos(3)*1.4   iPos(4)];
      |         end
      |     end
      | end
      mask TypeOptions QV: Voltage Control | Reactive Power Control
      mask TypeOptions LFpopup: Swing | PQ | PV
      mask Callback LFpopup:
      | % Get the mask parameter values. This is a cell
      | %   array of character vectors.
      | maskStr = get_param(gcb,'LFpopup');
      | p=Simulink.Mask.get(gcb);
      | 
      | % The pop-up menu is the first mask parameter.
      | %   Check the value selected in the pop-up
      | if strcmp(maskStr,'Swing'),
      | 
      |     % Set the visibility of both parameters on when
      |     %   User-defined is selected in the pop-up.
      |     p.getParameter('P0').Visible='off';
      |     p.getParameter('Q0').Visible='off';
      |     p.getParameter('V0').Visible='on';
      |     p.getParameter('Theta0').Visible='on';
      |     set_param([gcb '/Source_For_LF'],'BusType','swing');
      | 
      | elseif strcmp(maskStr,'PQ'),
      | 
      |     % Set the visibility of both parameters on when
      |     %   User-defined is selected in the pop-up.
      |     p.getParameter('P0').Visible='on';
      |     p.getParameter('Q0').Visible='on';
      |     p.getParameter('V0').Visible='off';
      |     p.getParameter('Theta0').Visible='off';
      |     set_param([gcb '/Source_For_LF'],'BusType','PQ');
      | 
      |     % Turn off the visibility of the Value field
      |     %   when User-defined is not selected.
      | else
      | 
      |     % Set the visibility of both parameters on when
      |     %   User-defined is selected in the pop-up.
      |     p.getParameter('P0').Visible='on';
      |     p.getParameter('Q0').Visible='off';
      |     p.getParameter('V0').Visible='on';
      |     p.getParameter('Theta0').Visible='off';
      |     set_param([gcb '/Source_For_LF'],'BusType','PV');
      | 
      | end
      mask DialogControl Container15 Prompt: Control gains
      mask DialogControl Container21 Prompt: LVRT
      mask DialogControl Control4 Prompt: Initial Operating Point
      mask DialogControl Container24 Prompt: VSC side
      mask DialogControl LF_vsc_str Prompt: V0 = 1.0108 pu, Angle = 0.4912°
      mask DialogControl Container25 Prompt: PCC
      mask DialogControl UpdateLoadflow Prompt: Update Loadflow
      mask DialogControl UpdateLoadflow Callback: LoadFlow_VSC
      mask Display:
      | x1=0.05;
      | y1=0.2;
      | %
      | plot([0.5 0.5]+x1,[0.97,0.8]-y1)
      | plot([0.5 0.32]+x1,[0.80 0.71]-y1)
      | plot([0.32 0.32]+x1,[0.80 0.52]-y1)
      | plot([0.32 0.5]+x1,[0.62 0.52]-y1)
      | plot([0.5 0.5]+x1,[0.52 0.35]-y1)
      | plot([0.45 0.5 0.43]+x1,[0.59 0.52 0.51]-y1)
      | %
      | plot([0.28 0.28]+x1,[0.74 0.58]-y1)
      | plot([0.28 0.20]+x1,[0.66 0.66]-y1)
      | %
      | plot([0.5 0.63]+x1,[0.84 0.84]-y1)
      | plot([0.63 0.63]+x1,[0.84 0.72]-y1)
      | plot([0.63 0.59]+x1,[0.72 0.65]-y1)
      | plot([0.63 0.67]+x1,[0.72 0.65]-y1)
      | plot([0.59 0.67]+x1,[0.65 0.65]-y1)
      | plot([0.63 0.63]+x1,[0.65 0.47]-y1)
      | plot([0.5 0.63]+x1,[0.47 0.47]-y1)
      | plot([0.58 0.67]+x1,[0.72 0.72]-y1)
      | %
      | color('blue')
      | text(0.3,0.10,'L-Filter GFL')
      | 
      | port_label('input',1,'\DeltaP (pu)','texmode','on');
      | port_label('input',2,'\DeltaQ (pu)','texmode','on');
      | port_label('output',1,'m');
      | port_label('rconn',1,'A');
      | port_label('rconn',2,'B');
      | port_label('rconn',3,'C');
      | port_label('lconn',1,'+');
      | port_label('lconn',2,'-');
  Mean Model 2-Level L-filter_old : Subsystem  Commented=on  mask(VSC){fn=50.0, Sn=1e9, Pn=1e9, Udcn=640e3, Output_Delay=375e-6, Un1=320e3, Un2=400e3, m=1, Rt_pu=0.005, Lt_pu=0.15, Lm_pu=inf, Rm_pu=inf, H_DC=0, wn_PLL=100, zeta_PLL=1, wn_i=1500, zeta_i=0.7, Kffi=on, Filtre_FF=off, w_ff=1000, QV=Reactive Power Control, w_P=10, w_V=50, w_LPF=4000, Imax=5, Iqmax=5, K_FRT=0, LFpopup=PQ, P0=0, Q0=0, V0=1.0108, Theta0=0.4912}
      mask prompts: fn "Nominal Frequency (Hz)"; Sn "Nominal Apparent Power (VA)"; Pn "Nominal Power (W)"; Udcn "Nominal DC Voltage (V)"; Output_Delay "Equivalent Ouput Delay (s)"; Un1 "VSC side Nominal Ph-Ph Voltage (V)"; Un2 "Grid side Nominal Ph-Ph Voltage (V)"; m "Transformer's ratio (p.u)"; Rt_pu "R (pu)"; Lt_pu "L (pu)"; Lm_pu "Rm (pu)"; Rm_pu "Lm (pu)"; H_DC "DC Inertia (ms)"; wn_PLL "Bandwidth (rad/s)"; zeta_PLL "Damping Ratio"; wn_i "Bandwidth (rad/s)"; zeta_i "Damping factor"; Kffi "Feedfoward Enable"; Filtre_FF "Filter of ff enable"; w_ff "Cutoff frequency (rad/s)"; QV "Mode"; w_P "Power control bandwidth"; w_V "Voltage control bandwidth"; w_LPF "Low-pass filters bandwidth"; Imax "Maximum current"; Iqmax "Maximum quadrature current"; K_FRT "LVRT block enabled (1) or disabled (0)"; P0 "Initial Active Power (pu)"; Q0 "Initial Reactive Power (pu)"; V0 "Initial Voltage (pu)"; Theta0 "Initial Angle (°)"
      mask init:
      | Init_Base;
      | Lc_eq = Lt_pu;
      | Init_LF_L;
      | Init_GFL;
      settings: OpenFcn=|
      | NameStr = get_param(gcb,'Name');
      | open_system(gcbh, 'Mask');
      | 
      | h2AllOpenDlgs = DAStudio.ToolRoot.getOpenDialogs;
      | 
      | for i=1:length(h2AllOpenDlgs)
      |     try
      |          %disp(h2AllOpenDlgs(i).getSource.getBlock.Name);
      |         Dialog_block_name = h2AllOpenDlgs(i).getSource.getBlock.Name;
      |          %strcmp(Dialog_block_name, NameStr),
      |         if (strcmp(h2AllOpenDlgs(i).getSource.getBlock.Name, NameStr))
      |             iPos = h2AllOpenDlgs(i).position;
      |             h2AllOpenDlgs(i).position = [iPos(1)   iPos(2)   iPos(3)*1.4   iPos(4)];
      |         end
      |     end
      | end
      mask TypeOptions QV: Voltage Control | Reactive Power Control
      mask TypeOptions LFpopup: Swing | PQ | PV
      mask Callback LFpopup:
      | % Get the mask parameter values. This is a cell
      | %   array of character vectors.
      | maskStr = get_param(gcb,'LFpopup');
      | p=Simulink.Mask.get(gcb);
      | 
      | % The pop-up menu is the first mask parameter.
      | %   Check the value selected in the pop-up
      | if strcmp(maskStr,'Swing'),
      | 
      |     % Set the visibility of both parameters on when
      |     %   User-defined is selected in the pop-up.
      |     p.getParameter('P0').Visible='off';
      |     p.getParameter('Q0').Visible='off';
      |     p.getParameter('V0').Visible='on';
      |     p.getParameter('Theta0').Visible='on';
      |     set_param([gcb '/Source_For_LF'],'BusType','swing');
      | 
      | elseif strcmp(maskStr,'PQ'),
      | 
      |     % Set the visibility of both parameters on when
      |     %   User-defined is selected in the pop-up.
      |     p.getParameter('P0').Visible='on';
      |     p.getParameter('Q0').Visible='on';
      |     p.getParameter('V0').Visible='off';
      |     p.getParameter('Theta0').Visible='off';
      |     set_param([gcb '/Source_For_LF'],'BusType','PQ');
      | 
      |     % Turn off the visibility of the Value field
      |     %   when User-defined is not selected.
      | else
      | 
      |     % Set the visibility of both parameters on when
      |     %   User-defined is selected in the pop-up.
      |     p.getParameter('P0').Visible='on';
      |     p.getParameter('Q0').Visible='off';
      |     p.getParameter('V0').Visible='on';
      |     p.getParameter('Theta0').Visible='off';
      |     set_param([gcb '/Source_For_LF'],'BusType','PV');
      | 
      | end
      mask DialogControl Container15 Prompt: Control gains
      mask DialogControl Container21 Prompt: LVRT
      mask DialogControl Control4 Prompt: Initial Operating Point
      mask DialogControl Container24 Prompt: VSC side
      mask DialogControl LF_vsc_str Prompt: V0 = 1.0108 pu, Angle = 0.4912°
      mask DialogControl Container25 Prompt: PCC
      mask DialogControl UpdateLoadflow Prompt: Update Loadflow
      mask DialogControl UpdateLoadflow Callback: LoadFlow_VSC
      mask Display:
      | x1=0.05;
      | y1=0.2;
      | %
      | plot([0.5 0.5]+x1,[0.97,0.8]-y1)
      | plot([0.5 0.32]+x1,[0.80 0.71]-y1)
      | plot([0.32 0.32]+x1,[0.80 0.52]-y1)
      | plot([0.32 0.5]+x1,[0.62 0.52]-y1)
      | plot([0.5 0.5]+x1,[0.52 0.35]-y1)
      | plot([0.45 0.5 0.43]+x1,[0.59 0.52 0.51]-y1)
      | %
      | plot([0.28 0.28]+x1,[0.74 0.58]-y1)
      | plot([0.28 0.20]+x1,[0.66 0.66]-y1)
      | %
      | plot([0.5 0.63]+x1,[0.84 0.84]-y1)
      | plot([0.63 0.63]+x1,[0.84 0.72]-y1)
      | plot([0.63 0.59]+x1,[0.72 0.65]-y1)
      | plot([0.63 0.67]+x1,[0.72 0.65]-y1)
      | plot([0.59 0.67]+x1,[0.65 0.65]-y1)
      | plot([0.63 0.63]+x1,[0.65 0.47]-y1)
      | plot([0.5 0.63]+x1,[0.47 0.47]-y1)
      | plot([0.58 0.67]+x1,[0.72 0.72]-y1)
      | %
      | color('blue')
      | text(0.3,0.10,'L-Filter GFL')
      | 
      | port_label('input',1,'\DeltaP (pu)','texmode','on');
      | port_label('input',2,'\DeltaQ (pu)','texmode','on');
      | port_label('output',1,'m');
      | port_label('rconn',1,'A');
      | port_label('rconn',2,'B');
      | port_label('rconn',3,'C');
      | port_label('lconn',1,'+');
      | port_label('lconn',2,'0');
      | port_label('lconn',3,'-');
  Mean Model 2-Level L-filter_sav : Subsystem  Commented=on  mask(VSC){fn=50, Sn=10e3, Pn=10e3, Udcn=750, Time_Step=50e-6, Un1=400, Un2=400, Rt_pu=0.005, Lt_pu=0.15, Lm_pu=500, Rm_pu=500, Tr_PLL=10e-3, Tr_i=1e-3, zeta_i=1, LFpopup=PQ, P0=0.5, Q0=1.2614e-05, V0=1.0015, Theta0=0.56166}
      mask prompts: fn "Nominal Frequency (Hz)"; Sn "Nominal Apparent Power (VA)"; Pn "Nominal Power (W)"; Udcn "Nominal DC Voltage (V)"; Time_Step "Sample Time (s)"; Un1 "VSC side Nominal Ph-Ph Voltage (V)"; Un2 "Grid side Nominal Ph-Ph Voltage (V)"; Rt_pu "R (pu)"; Lt_pu "L (pu)"; Lm_pu "Rm (pu)"; Rm_pu "Lm (pu)"; Tr_PLL "Time response (ms)"; Tr_i "Time response (s)"; zeta_i "Damping Factor"; P0 "Initial Active Power (pu)"; Q0 "Initial Reactive Power (pu)"; V0 "Initial Voltage (pu)"; Theta0 "Initial Angle (°)"
      mask init:
      | % Update Name of LF bus for internal purpose
      |     NameStr = [get_param(gcb,'Name')];% '_LF'];
      |     set_param([gcb '/Load Flow Bus'],'ID',NameStr);    
      |     
      | % Base values
      |     fb = fn;
      |     Pb = Pn;
      |     cos_phi_n = Pn/Sn;
      |     Sb = Pb/cos_phi_n;
      |     Vn1 = Un1/sqrt(3);
      |     Vb1 = Vn1;
      |     Vn2 = Un2/sqrt(3);
      |     Vb2 = Vn2;
      |     Ib1 = Sb / 3*Vb1;
      |     Ib2 = Sb / (3*Vb2);
      |     wb = 2*pi*fb;
      |     
      | % current control tuning
      |     Lf_pu = Lt_pu;
      |     Rf_pu = Rt_pu;
      |     wn_i = 3/Tr_i;
      |     Kp_i = 2*zeta_i*wn_i*Lf_pu/wb-Rf_pu;
      |     Ti_i = 2*zeta_i/wn_i-Rf_pu/(wn_i^2*Lf_pu/wb);
      |     Ki_i = Kp_i/Ti_i;
      |     Kffi = 1;
      |     
      | % Compute the delay compensation between control and power parts
      |     if (Time_Step == -1)
      |         Solver_Time_Step = 0;
      |     else
      |         Solver_Time_Step = Time_Step;
      |     end
      | 
      | % Compute Initial Voltage of VSC 
      | %   from steady-state output transformer model and Loadflow result
      |     
      |     %Initialize correctly the LoadFlow bus parameters connected to PCC
      |     VLF = V0;
      |     ThetaLF = Theta0;
      |     if (LFpopup == 'PQ')
      |         VLF = 1;
      |         ThetaLF = 0;
      |     elseif (LFpopup == 'PV')
      |         VLF = V0;
      |         ThetaLF = 0;        
      |     end
      |     set_param([gcb '/Load Flow Bus'],'Vref',num2str(VLF),'Vangle',num2str(ThetaLF));
      |     
      |     R1_pu = Rt_pu/2;
      |     L1_pu = Lt_pu/2;
      |     R2_pu = Rt_pu/2;
      |     L2_pu = Lt_pu/2;
      |     X1_pu = L1_pu;
      |     X2_pu = L2_pu;
      |     Xm_pu = Lm_pu;
      |     
      |     Zm_pu = 1/(1/Rm_pu+1/(1i*Xm_pu));
      | 
      |     S0=P0+1i*Q0;
      |     I2 = conj(S0)/(V0);
      | 
      |     Vm = (R2_pu+1i*X2_pu)*I2 + V0;
      |     Im = Vm/Zm_pu;
      | 
      |     I1 = I2 + Im;
      |     V1 = (R1_pu+1i*X1_pu) * I1 + Vm;
      | 
      |     Vvsc0 = abs(V1);
      |     Theta_vsc0 = angle(V1) * 180/pi+Theta0;
      |     
      |     Va0 = Vvsc0*sqrt(2)*Vb1*sin(Theta_vsc0*pi/180);
      |     Vb0 = Vvsc0*sqrt(2)*Vb1*sin(Theta_vsc0*pi/180-2*pi/3);
      |     Vc0 = Vvsc0*sqrt(2)*Vb1*sin(Theta_vsc0*pi/180+2*pi/3);
      |     
      |     Vm0_d = Vvsc0*cos(angle(V1));
      |     Vm0_q = Vvsc0*sin(angle(V1));
      |     
      | % Generate string to display LF results on Mask
      |     %str_tmp = fprintf("Vvsc0 = %d, Theta_vsc0 = %d°",Vvsc0,Theta_vsc0);
      |     mo = get_param(gcb,'MaskObject');
      |     mo.getDialogControl('LF_vsc_str').Prompt = ['V0 = ', num2str(Vvsc0),' pu, Angle = ', num2str(Theta_vsc0),'°'];
      |     mo.getDialogControl('LF_pcc_str').Prompt = ['V0 = ', num2str(V0),' pu, Angle = ', num2str(Theta0),'°'];
      |     mo.getDialogControl('LF_pcc_Power_str').Prompt = ['P0 = ', num2str(P0),' pu, Q0 = ', num2str(Q0),' pu'];
      |     %set_param([gcb],'LF_str',str_tmp);
      settings: OpenFcn=|
      | NameStr = get_param(gcb,'Name');
      | open_system(gcbh, 'Mask');
      | 
      | h2AllOpenDlgs = DAStudio.ToolRoot.getOpenDialogs;
      | 
      | for i=1:length(h2AllOpenDlgs)
      |     try
      |          %disp(h2AllOpenDlgs(i).getSource.getBlock.Name);
      |         Dialog_block_name = h2AllOpenDlgs(i).getSource.getBlock.Name;
      |          %strcmp(Dialog_block_name, NameStr),
      |         if (strcmp(h2AllOpenDlgs(i).getSource.getBlock.Name, NameStr))
      |             iPos = h2AllOpenDlgs(i).position;
      |             h2AllOpenDlgs(i).position = [iPos(1)   iPos(2)   iPos(3)*1.4   iPos(4)];
      |         end
      |     end
      | end
      mask TypeOptions LFpopup: Swing | PQ | PV
      mask Callback LFpopup:
      | % Get the mask parameter values. This is a cell
      | %   array of character vectors.
      | maskStr = get_param(gcb,'LFpopup');
      | p=Simulink.Mask.get(gcb);
      | 
      | % The pop-up menu is the first mask parameter.
      | %   Check the value selected in the pop-up
      | if strcmp(maskStr,'Swing'),
      | 
      |     % Set the visibility of both parameters on when
      |     %   User-defined is selected in the pop-up.
      |     p.getParameter('P0').Visible='off';
      |     p.getParameter('Q0').Visible='off';
      |     p.getParameter('V0').Visible='on';
      |     p.getParameter('Theta0').Visible='on';
      |     set_param([gcb '/Source_For_LF'],'BusType','swing');
      | 
      | elseif strcmp(maskStr,'PQ'),
      | 
      |     % Set the visibility of both parameters on when
      |     %   User-defined is selected in the pop-up.
      |     p.getParameter('P0').Visible='on';
      |     p.getParameter('Q0').Visible='on';
      |     p.getParameter('V0').Visible='off';
      |     p.getParameter('Theta0').Visible='off';
      |     set_param([gcb '/Source_For_LF'],'BusType','PQ');
      | 
      |     % Turn off the visibility of the Value field
      |     %   when User-defined is not selected.
      | else
      | 
      |     % Set the visibility of both parameters on when
      |     %   User-defined is selected in the pop-up.
      |     p.getParameter('P0').Visible='on';
      |     p.getParameter('Q0').Visible='off';
      |     p.getParameter('V0').Visible='on';
      |     p.getParameter('Theta0').Visible='off';
      |     set_param([gcb '/Source_For_LF'],'BusType','PV');
      | 
      | end
      mask DialogControl Control4 Prompt: Initial Operating Point
      mask DialogControl Container24 Prompt: VSC side
      mask DialogControl LF_vsc_str Prompt: V0 = 1.0069 pu, Angle = 4.8354°
      mask DialogControl Container25 Prompt: PCC
      mask DialogControl UpdateLoadflow Prompt: Update Loadflow
      mask DialogControl UpdateLoadflow Callback: LoadFlow_VSC
      mask Display:
      | disp('Grid-Feeding\n\n');
      | disp('\nL-Filter');
      | port_label('input',1,'dE_set (pu)');
      | port_label('input',2,'dP_set (pu)');
      | port_label('output',1,'m');
      | port_label('rconn',1,'A');
      | port_label('rconn',2,'B');
      | port_label('rconn',3,'C');
  Mean Model 2-Level LCL-filter [under construction] : Subsystem  Commented=on  mask(VSC){fn=50, Sn=10e3, Pn=10e3, Udcn=750, Un1=400, Un2=400, Rt_pu=0.005, Lt_pu=0.15, Lm_pu=500, Rm_pu=500, Tr_PLL=10e-3, Tr_i=1e-3, zeta_i=1, LFpopup=PQ, P0=0.5, Q0=1.2614e-05, V0=1.0015, Theta0=0.56166}
      mask prompts: fn "Nominal Frequency (Hz)"; Sn "Nominal Apparent Power (VA)"; Pn "Nominal Power (W)"; Udcn "Nominal DC Voltage (V)"; Un1 "VSC side Nominal Ph-Ph Voltage (V)"; Un2 "Grid side Nominal Ph-Ph Voltage (V)"; Rt_pu "R (pu)"; Lt_pu "L (pu)"; Lm_pu "Rm (pu)"; Rm_pu "Lm (pu)"; Tr_PLL "Time response (s)"; Tr_i "Time response (s)"; zeta_i "Damping Factor"; P0 "Initial Active Power (pu)"; Q0 "Initial Reactive Power (pu)"; V0 "Initial Voltage (pu)"; Theta0 "Initial Angle (°)"
      mask init:
      | % Update Name of LF bus for internal purpose
      |     NameStr = [get_param(gcb,'Name')];% '_LF'];
      |     set_param([gcb '/Load Flow Bus'],'ID',NameStr);    
      |     
      | % Base values
      |     fb = fn;
      |     Pb = Pn;
      |     cos_phi_n = Pn/Sn;
      |     Sb = Pb/cos_phi_n;
      |     Vn1 = Un1/sqrt(3);
      |     Vb1 = Vn1;
      |     Vn2 = Un2/sqrt(3);
      |     Vb2 = Vn2;
      |     Ib1 = Sb / 3*Vb1;
      |     Ib2 = Sb / (3*Vb2);
      |     wb = 2*pi*fb;
      |   
      | % PLL derivation of the parameters
      |     %wn_PLL=5/Tr_PLL;
      |     %zeta_PLL = 1;
      |     %Kp_PLL_pu = 2*zeta_PLL*wn_PLL/wb;
      |     %Ki_PLL_pu = wn_PLL^2/wb;
      |     
      | % current control tuning
      |     Lf_pu = Lt_pu;
      |     Rf_pu = Rt_pu;
      |     wn_i = 3/Tr_i;
      |     Kp_i = 2*zeta_i*wn_i*Lf_pu/wb-Rf_pu;
      |     Ti_i = 2*zeta_i/wn_i-Rf_pu/(wn_i^2*Lf_pu/wb);
      |     Ki_i = Kp_i/Ti_i;
      |     Kffi = 1;
      | 
      | 
      | % Compute Initial Voltage of VSC 
      | %   from steady-state output transformer model and Loadflow result
      |     
      |     %Initialize correctly the LoadFlow bus parameters connected to PCC
      |     VLF = V0;
      |     ThetaLF = Theta0;
      |     if (LFpopup == 'PQ')
      |         VLF = 1;
      |         ThetaLF = 0;
      |     elseif (LFpopup == 'PV')
      |         VLF = V0;
      |         ThetaLF = 0;        
      |     end
      |     set_param([gcb '/Load Flow Bus'],'Vref',num2str(VLF),'Vangle',num2str(ThetaLF));
      |     
      |     R1_pu = Rt_pu/2;
      |     L1_pu = Lt_pu/2;
      |     R2_pu = Rt_pu/2;
      |     L2_pu = Lt_pu/2;
      |     X1_pu = L1_pu;
      |     X2_pu = L2_pu;
      |     Xm_pu = Lm_pu;
      |     
      |     Zm_pu = 1/(1/Rm_pu+1/(1i*Xm_pu));
      | 
      |     S0=P0+1i*Q0;
      |     I2 = conj(S0)/(V0);
      | 
      |     Vm = (R2_pu+1i*X2_pu)*I2 + V0;
      |     Im = Vm/Zm_pu;
      | 
      |     I1 = I2 + Im;
      |     V1 = (R1_pu+1i*X1_pu) * I1 + Vm;
      | 
      |     Vvsc0 = abs(V1);
      |     Theta_vsc0 = angle(V1) * 180/pi+Theta0;
      |     
      |     Va0 = Vvsc0*sqrt(2)*Vb1*sin(Theta_vsc0*pi/180);
      |     Vb0 = Vvsc0*sqrt(2)*Vb1*sin(Theta_vsc0*pi/180-2*pi/3);
      |     Vc0 = Vvsc0*sqrt(2)*Vb1*sin(Theta_vsc0*pi/180+2*pi/3);
      |     
      |     Vm0_d = Vvsc0*cos(angle(V1));
      |     Vm0_q = Vvsc0*sin(angle(V1));
      |     
      | % Generate string to display LF results on Mask
      |     %str_tmp = fprintf("Vvsc0 = %d, Theta_vsc0 = %d°",Vvsc0,Theta_vsc0);
      |     mo = get_param(gcb,'MaskObject');
      |     mo.getDialogControl('LF_vsc_str').Prompt = ['V0 = ', num2str(Vvsc0),' pu, Angle = ', num2str(Theta_vsc0),'°'];
      |     mo.getDialogControl('LF_pcc_str').Prompt = ['V0 = ', num2str(V0),' pu, Angle = ', num2str(Theta0),'°'];
      |     mo.getDialogControl('LF_pcc_Power_str').Prompt = ['P0 = ', num2str(P0),' pu, Q0 = ', num2str(Q0),' pu'];
      |     %set_param([gcb],'LF_str',str_tmp);
      settings: OpenFcn=|
      | NameStr = get_param(gcb,'Name');
      | open_system(gcbh, 'Mask');
      | 
      | h2AllOpenDlgs = DAStudio.ToolRoot.getOpenDialogs;
      | 
      | for i=1:length(h2AllOpenDlgs)
      |     try
      |          %disp(h2AllOpenDlgs(i).getSource.getBlock.Name);
      |         Dialog_block_name = h2AllOpenDlgs(i).getSource.getBlock.Name;
      |          %strcmp(Dialog_block_name, NameStr),
      |         if (strcmp(h2AllOpenDlgs(i).getSource.getBlock.Name, NameStr))
      |             iPos = h2AllOpenDlgs(i).position;
      |             h2AllOpenDlgs(i).position = [iPos(1)   iPos(2)   iPos(3)*1.4   iPos(4)];
      |         end
      |     end
      | end
      mask TypeOptions LFpopup: Swing | PQ | PV
      mask Callback LFpopup:
      | % Get the mask parameter values. This is a cell
      | %   array of character vectors.
      | maskStr = get_param(gcb,'LFpopup');
      | p=Simulink.Mask.get(gcb);
      | 
      | % The pop-up menu is the first mask parameter.
      | %   Check the value selected in the pop-up
      | if strcmp(maskStr,'Swing'),
      | 
      |     % Set the visibility of both parameters on when
      |     %   User-defined is selected in the pop-up.
      |     p.getParameter('P0').Visible='off';
      |     p.getParameter('Q0').Visible='off';
      |     p.getParameter('V0').Visible='on';
      |     p.getParameter('Theta0').Visible='on';
      |     set_param([gcb '/Source_For_LF'],'BusType','swing');
      | 
      | elseif strcmp(maskStr,'PQ'),
      | 
      |     % Set the visibility of both parameters on when
      |     %   User-defined is selected in the pop-up.
      |     p.getParameter('P0').Visible='on';
      |     p.getParameter('Q0').Visible='on';
      |     p.getParameter('V0').Visible='off';
      |     p.getParameter('Theta0').Visible='off';
      |     set_param([gcb '/Source_For_LF'],'BusType','PQ');
      | 
      |     % Turn off the visibility of the Value field
      |     %   when User-defined is not selected.
      | else
      | 
      |     % Set the visibility of both parameters on when
      |     %   User-defined is selected in the pop-up.
      |     p.getParameter('P0').Visible='on';
      |     p.getParameter('Q0').Visible='off';
      |     p.getParameter('V0').Visible='on';
      |     p.getParameter('Theta0').Visible='off';
      |     set_param([gcb '/Source_For_LF'],'BusType','PV');
      | 
      | end
      mask DialogControl Control4 Prompt: Initial Operating Point
      mask DialogControl Container24 Prompt: VSC side
      mask DialogControl LF_vsc_str Prompt: V0 = 1.0069 pu, Angle = 4.8354°
      mask DialogControl Container25 Prompt: PCC
      mask DialogControl UpdateLoadflow Prompt: Update Loadflow
      mask DialogControl UpdateLoadflow Callback: LoadFlow_VSC
      mask Display:
      | disp('Grid-Feeding\n\n');
      | disp('\nL-Filter');
      | port_label('input',1,'dE_set (pu)');
      | port_label('input',2,'dP_set (pu)');
      | port_label('output',1,'m');
      | port_label('rconn',1,'A');
      | port_label('rconn',2,'B');
      | port_label('rconn',3,'C');
